simulink model "STLA_8_31"  (R2020b)
settings: Solver=ode3  StartTime=0.0  StopTime=2474  FixedStep=0.01  RelTol=1e-3
model workspace (MAT data in the model file):
  qw = 0.5
undefined symbols (not defined in the file): BSFC, continuous_torque_M, eff_speeds, eff_torques, h, km, m, m_eff, Padd, peak_torque_M, pedal_Brake, pedal_Comfort, pedal_ECO, pedal_Sport, rpm_E, rpm_M, s, speed_bp, speed_Brake, speed_Comfort, speed_ECO, speed_Sport, Tmax_eng, Topt_eng, torque_bp, torque_Brake, Torque_BSFC, torque_Comfort, torque_ECO, torque_Sport
libraries: simulink x12, svdutilitieslib x2, instrumentlib x2, autolibshared x1, aerolibconvert2 x1, pid_lib x1
(part 1 of 2)
settings Model: Creator=王刚  LastModifiedBy=王刚
settings DebuggingCC: UnconnectedInputMsg=none  UnconnectedOutputMsg=none  UnconnectedLineMsg=none
settings ModelReferenceCC: EnableRefExpFcnMdlSchedulingChecks=off
settings RTWCC: GPUComputeCapability=5.0
settings ConfigComp: CovBoundaryAbsTol=1.0e-5

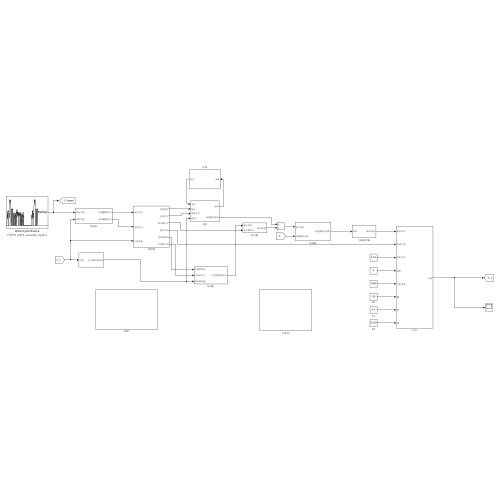
[thumbnail: Simulink's stored preview of the top-level diagram]
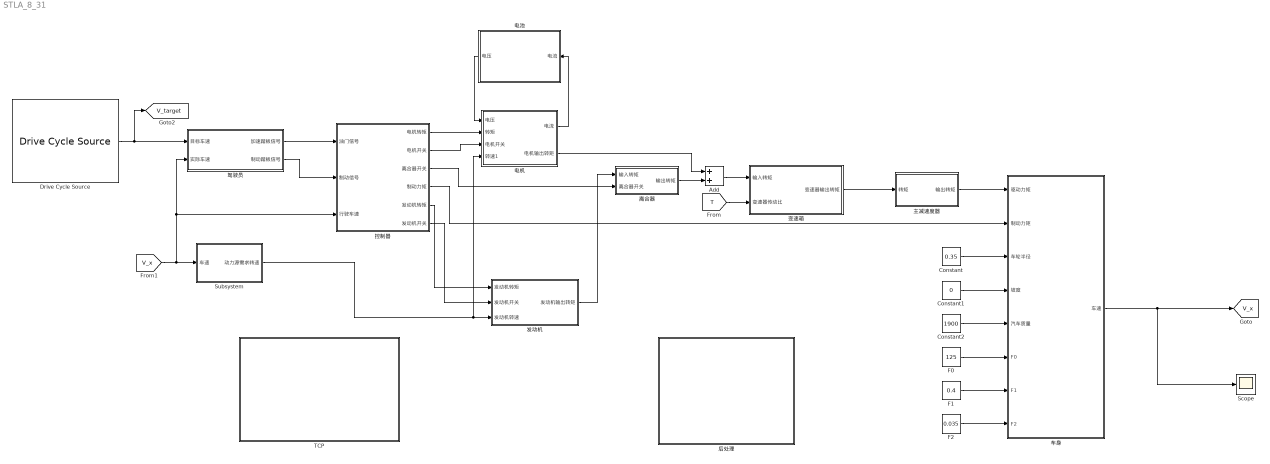
== system STLA_8_31 ==
  Add : Sum
  Constant : Constant  Value=0.35
  Constant1 : Constant  Value=0
  Constant2 : Constant  Value=1900
  Drive Cycle Source : autolibshared/Drive Cycle Source  cycleVar=FTP75  fileVar=cycleFTP75.mat  tfinal="2474  seconds, Cyclic"  cycleRepeat=on  outAccPort=off  outGearPort=off  gearList=No gear data  t_wot1=5  xdot_woto=0  xdot_wot1=30  t_wot2=20  xdot_wot2=0  t_wotend=30  srcUnit=m/s  outUnit=km/h  srcAccUnit=m/s/s  outAccUnit=m/s^2  dt=0  aMode=1  faultOption=off  velBnd=2  velBndUnit=mph  inUnit=m/s  timeBnd=1  failOption=off  stopSim=off  maxFaultCnt=10  maxFaultTime=2  maxTotFaultTime=15  traceOption=off  dtTrace=1  traceWindow=10  lastDCname=FTP75  lastOutUnit=mph  lastDT=0  lastTB=1  lastSB=2  forceCalcBound=off
  F0 : Constant  Value=125
  F1 : Constant  Value=0.4
  F2 : Constant  Value=0.035
  Scope : Scope
  Subsystem : Subsystem
  TCP : Subsystem
  主减速度器 : Subsystem
  发动机 : Subsystem
  变速箱 : Subsystem
  后处理 : Subsystem
  控制器 : Subsystem
  电机 : Subsystem
  电池 : Subsystem
  离合器 : Subsystem
  车身 : Subsystem
  驾驶员 : Subsystem
  tag scope: V_target=global, V_x=global
  wires:
  驾驶员/1(加速踏板信号) -> 控制器/1(油门信号)
  驾驶员/2(制动踏板信号) -> 控制器/2(制动信号)
  Constant/1 -> 车身/3(车轮半径)
  Constant1/1 -> 车身/4(坡度)
  Constant2/1 -> 车身/5(汽车质量)
  F0/1 -> 车身/6(F0)
  F1/1 -> 车身/7(F1)
  F2/1 -> 车身/8(F2)
  变速箱/1(变速器输出转矩) -> 主减速度器/1(转矩)
  主减速度器/1(输出转矩) -> 车身/1("驱动力矩 ")
  控制器/5(发动机转矩) -> 发动机/1(发动机转矩)
  控制器/6(发动机开关) -> 发动机/2(发动机开关)
  控制器/1(电机转矩) -> 电机/2(转矩)
  控制器/2(电机开关) -> 电机/3(电机开关)
  控制器/3(离合器开关) -> 离合器/2(离合器开关)
  控制器/4(制动力矩) -> 车身/2(" 制动力矩")
  电池/1(电压) -> 电机/1(电压)
  离合器/1(输出转矩) -> Add/2
  Add/1 -> 变速箱/1(输入转矩)
  [T] -> 变速箱/2(变速器传动比)
  车身/1(车速) -> [V_x], Scope/1
  [V_x] -> 驾驶员/2(实际车速), 控制器/3(行驶车速), Subsystem/1(车速)
  电机/1(电流) -> 电池/1(电流)
  电机/2(电机输出转矩) -> Add/1
  发动机/1(发动机输出转矩) -> 离合器/1(输入转矩)
  Subsystem/1(动力源需求转速) -> 电机/4(转速1), 发动机/3(发动机转速)
  Drive Cycle Source/1 -> [V_target], 驾驶员/1(目标车速)

== system STLA_8_31/Subsystem ==
  车速 : Inport
  " " : Constant  Value=0.377
  Product : Product  Inputs=***//
  主减速器传动比 : Constant  Value=4.88
  车轮半径 : Constant  Value=0.25
  动力源需求转速 : Outport
  tag scope: rmp=global
  wires:
  Product/1 -> [rmp], 动力源需求转速/1
  车速/1 -> Product/1
  " "/1 -> Product/5
  主减速器传动比/1 -> Product/2
  车轮半径/1 -> Product/4
  [T] -> Product/3

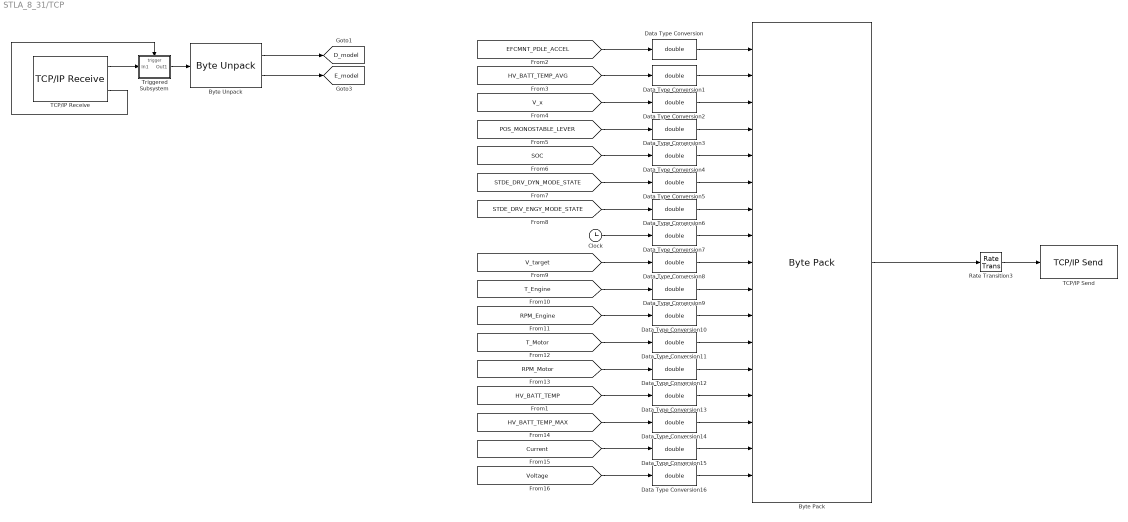
== system STLA_8_31/TCP ==
  Byte Pack : svdutilitieslib/Byte Pack  maskPackedDataType=uint8  datatypes={'double', 'double', 'double', 'double', 'double', 'double', 'double', 'double', 'double', 'double', 'double', 'double', 'double', 'double', 'double', 'double', 'double'}  byteAlign=1  blockPlatform=tic2000
  Byte Unpack : svdutilitieslib/Byte Unpack  dimensions={[1] [1]}  datatypes={'double', 'double'}  byteAlign=1  blockPlatform=tic2000
  Clock : Clock
  Data Type Conversion{,1..16} (17 alike) : DataTypeConversion  OutDataTypeStr=double
  Rate Transition3 : RateTransition  OutPortSampleTime=0.1
  TCP/IP Receive : instrumentlib/TCP//IP Receive  Host=127.0.0.1  Port=5000  DataSize=16  DataType=uint8  ASCIIFormatting=%f  Terminator=LF  ByteOrder=LittleEndian  EnableBlockingMode=off  Timeout=0.01  SampleTime=0.01
  TCP/IP Send : instrumentlib/TCP//IP Send  Host=127.0.0.1  Port=5001  ByteOrder=LittleEndian  EnableBlockingMode=off  Timeout=10  TransferDelay=on
  Triggered Subsystem : Subsystem  TreatAsAtomicUnit=on
  tag scope: D_model=global, E_model=global
  wires:
  [SOC] -> Data Type Conversion4/1
  [V_x] -> Data Type Conversion2/1
  Byte Unpack/2 -> [E_model]
  Data Type Conversion1/1 -> Byte Pack/2
  Data Type Conversion8/1 -> Byte Pack/9
  Data Type Conversion6/1 -> Byte Pack/7
  [V_target] -> Data Type Conversion8/1
  [EFCMNT_PDLE_ACCEL] -> Data Type Conversion/1
  [RPM_Engine] -> Data Type Conversion10/1
  [STDE_DRV_DYN_MODE_STATE] -> Data Type Conversion5/1
  Data Type Conversion12/1 -> Byte Pack/13
  Data Type Conversion3/1 -> Byte Pack/4
  [T_Engine] -> Data Type Conversion9/1
  Data Type Conversion10/1 -> Byte Pack/11
  Data Type Conversion5/1 -> Byte Pack/6
  Data Type Conversion11/1 -> Byte Pack/12
  Byte Pack/1 -> Rate Transition3/1
  TCP/IP Receive/2 -> Triggered Subsystem/Trigger
  TCP/IP Receive/1 -> Triggered Subsystem/1(In1)
  [T_Motor] -> Data Type Conversion11/1
  Triggered Subsystem/1(Out1) -> Byte Unpack/1
  Data Type Conversion4/1 -> Byte Pack/5
  Byte Unpack/1 -> [D_model]
  [POS_MONOSTABLE_LEVER] -> Data Type Conversion3/1
  [RPM_Motor] -> Data Type Conversion12/1
  Data Type Conversion2/1 -> Byte Pack/3
  [STDE_DRV_ENGY_MODE_STATE] -> Data Type Conversion6/1
  Clock/1 -> Data Type Conversion7/1
  Data Type Conversion7/1 -> Byte Pack/8
  Rate Transition3/1 -> TCP/IP Send/1
  [HV_BATT_TEMP_AVG] -> Data Type Conversion1/1
  Data Type Conversion9/1 -> Byte Pack/10
  Data Type Conversion/1 -> Byte Pack/1
  [HV_BATT_TEMP] -> Data Type Conversion13/1
  [HV_BATT_TEMP_MAX] -> Data Type Conversion14/1
  Data Type Conversion13/1 -> Byte Pack/14
  Data Type Conversion14/1 -> Byte Pack/15
  [Current] -> Data Type Conversion15/1
  [Voltage] -> Data Type Conversion16/1
  Data Type Conversion15/1 -> Byte Pack/16
  Data Type Conversion16/1 -> Byte Pack/17

== system STLA_8_31/主减速度器 ==
  转矩 : Inport
  Product : Product
  主减速器传动比 : Constant  Value=4.88
  传动效率 : Gain  Gain=0.9
  输出转矩 : Outport
  wires:
  转矩/1 -> Product/1
  主减速器传动比/1 -> Product/2
  Product/1 -> 传动效率/1
  传动效率/1 -> 输出转矩/1

== system STLA_8_31/发动机 ==
  发动机转矩 : Inport
  发动机开关 : Inport  Port=2
  发动机转速 : Inport  Port=3
  2-D Lookup Table : Lookup_n-D  BreakpointsForDimension1=Torque_BSFC  BreakpointsForDimension2=rpm_E  Table=BSFC  InternalRulePriority=Speed  RndMeth=Simplest  InputSameDT=on
      settings: InputPortMap=u0,u1
  Constant : Constant  Value=9550
  Constant1 : Constant  Value=3600
  Gain : Gain  Gain=-1
  Integrator : Integrator
  Product : Product
  Product1 : Product  Inputs=***/
  Product2 : Product  Inputs=**/
  Product3 : Product
  Saturation Dynamic : simulink/Discontinuities/Saturation Dynamic  OutMin=[]  OutMax=[]  OutDataTypeStr=Inherit: Same as second input  OutDataType=fixdt(1, 16)  OutScaling=2^-10  DoSatur=off
  Scope : Scope
  Scope2 : Scope  NumInputPorts=3
  Scope3 : Scope  NumInputPorts=2
  外特性 : Lookup_n-D  NumberOfTableDimensions=1  BreakpointsForDimension1=rpm_E  Table=Tmax_eng  InternalRulePriority=Speed  RndMeth=Simplest  InputSameDT=on
  最优转矩 : Lookup_n-D  NumberOfTableDimensions=1  BreakpointsForDimension1=rpm_E  Table=Topt_eng  InternalRulePriority=Speed  RndMeth=Simplest  InputSameDT=on
  发动机输出转矩 : Outport
  tag scope: M_f=global, RPM_Engine=global, T_Engine=global, Te_max=global, Te_opt=global
  wires:
  Constant/1 -> Product1/4
  Product1/1 -> Product2/1, Scope/1
  发动机开关/1 -> Product3/2, Product1/3, Scope2/2, Product/1
  最优转矩/1 -> Scope3/2, [Te_opt]
  外特性/1 -> Gain/1, Scope3/1, Saturation Dynamic/1, [Te_max]
  发动机转矩/1 -> 2-D Lookup Table/1, Product1/2, Scope2/3, Product/2
  Saturation Dynamic/1 -> Scope2/1, 发动机输出转矩/1, [T_Engine]
  Product/1 -> Saturation Dynamic/2
  Gain/1 -> Saturation Dynamic/3
  2-D Lookup Table/1 -> Product2/2
  Constant1/1 -> Product2/3
  Product2/1 -> Integrator/1
  Integrator/1 -> [M_f]
  发动机转速/1 -> Product3/1, 最优转矩/1, 2-D Lookup Table/2, Product1/1, 外特性/1
  Product3/1 -> [RPM_Engine]

== system STLA_8_31/变速箱 ==
  输入转矩 : Inport
  变速器传动比 : Inport  Port=2
  Product : Product
  变速器输出转矩 : Outport
  wires:
  输入转矩/1 -> Product/1
  变速器传动比/1 -> Product/2
  Product/1 -> 变速器输出转矩/1

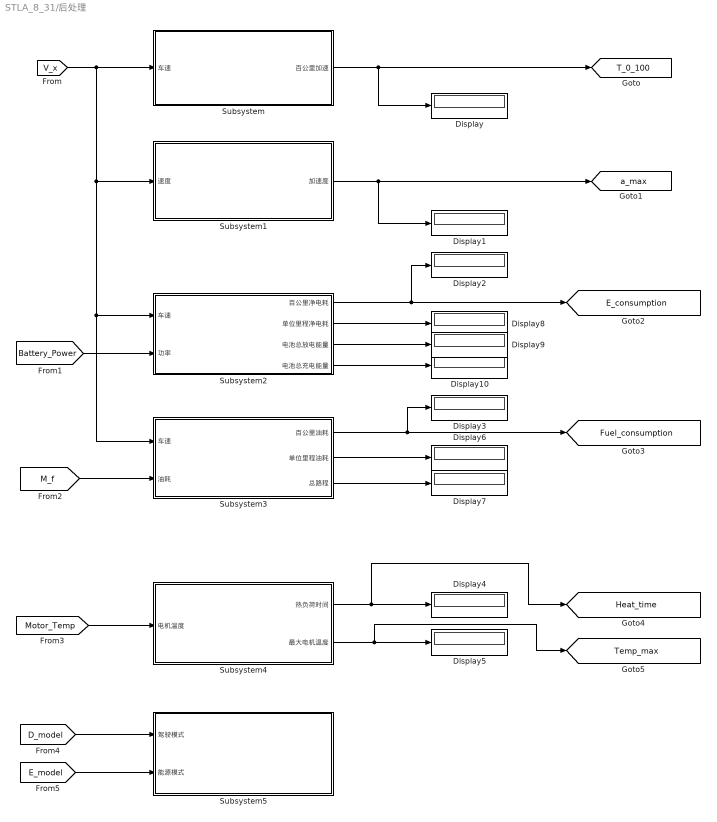
== system STLA_8_31/后处理 ==
  Display{,1..10} (11 alike) : Display
  Subsystem : Subsystem
  Subsystem1 : Subsystem
  Subsystem2 : Subsystem
  Subsystem3 : Subsystem
  Subsystem4 : Subsystem
  Subsystem5 : Subsystem
  tag scope: E_consumption=global, Fuel_consumption=global, Heat_time=global, T_0_100=global, Temp_max=global, a_max=global
  wires:
  [V_x] -> Subsystem2/1(车速), Subsystem3/1(车速), Subsystem1/1(速度), Subsystem/1(车速)
  Subsystem2/1(百公里净电耗) -> Display2/1, [E_consumption]
  [Battery_Power] -> Subsystem2/2(功率)
  [M_f] -> Subsystem3/2(油耗)
  Subsystem3/1(百公里油耗) -> [Fuel_consumption], Display3/1
  [Motor_Temp] -> Subsystem4/1(电机温度)
  Subsystem4/1(热负荷时间) -> [Heat_time], Display4/1
  [D_model] -> Subsystem5/1(驾驶模式)
  Subsystem/1(百公里加速) -> Display/1, [T_0_100]
  Subsystem1/1(加速度) -> Display1/1, [a_max]
  Subsystem4/2(最大电机温度) -> [Temp_max], Display5/1
  [E_model] -> Subsystem5/2(能源模式)
  Subsystem3/2(单位里程油耗) -> Display6/1
  Subsystem3/3(总路程) -> Display7/1
  Subsystem2/2(单位里程净电耗) -> Display8/1
  Subsystem2/3(电池总放电能量) -> Display9/1
  Subsystem2/4(电池总充电能量) -> Display10/1

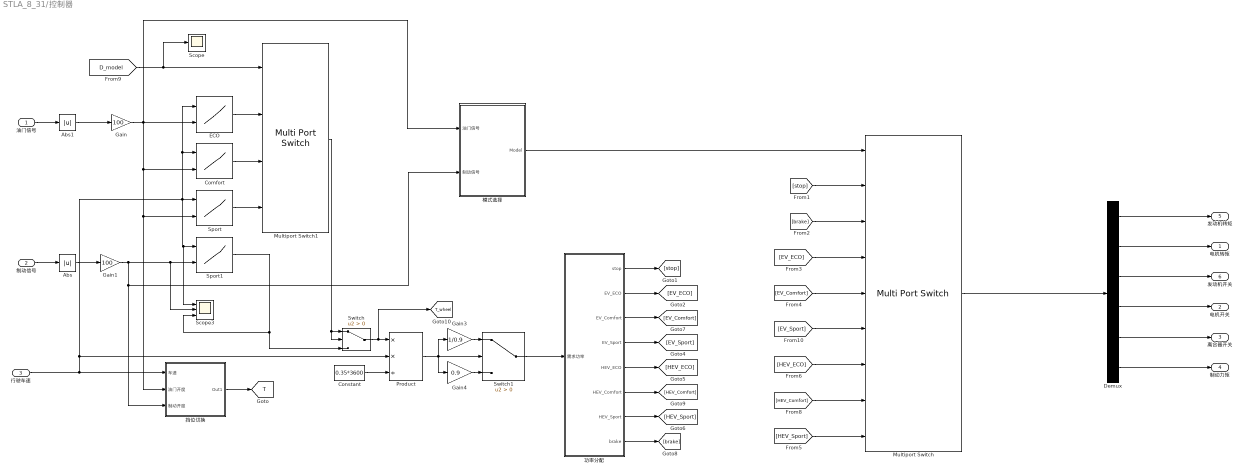
== system STLA_8_31/控制器 ==
  油门信号 : Inport
  制动信号 : Inport  Port=2
  行驶车速 : Inport  Port=3
  Abs : Abs  ZeroCross=off
  Abs1 : Abs  ZeroCross=off
  Comfort : Lookup_n-D  BreakpointsForDimension1=speed_Comfort  BreakpointsForDimension2=pedal_Comfort  Table=torque_Comfort  InternalRulePriority=Speed  RndMeth=Simplest  InputSameDT=on
      settings: InputPortMap=u0,u1
  Constant : Constant  Value=0.35*3600
  Demux : Demux  Outputs=6
  ECO : Lookup_n-D  BreakpointsForDimension1=speed_ECO  BreakpointsForDimension2=pedal_ECO  Table=torque_ECO  InternalRulePriority=Speed  RndMeth=Simplest  InputSameDT=on
      settings: InputPortMap=u0,u1
  Gain : Gain  Gain=100
  Gain1 : Gain  Gain=100
  Gain3 : Gain  Gain=1/0.9
  Gain4 : Gain  Gain=0.9
  Multiport Switch : MultiPortSwitch  Inputs=8
  Multiport Switch1 : MultiPortSwitch  DataPortOrder=Zero-based contiguous  DiagnosticForDefault=None  zeroidx=on
  Product : Product  Inputs=**/
  Scope : Scope
  Scope3 : Scope  NumInputPorts=3
  Sport : Lookup_n-D  BreakpointsForDimension1=speed_Sport  BreakpointsForDimension2=pedal_Sport  Table=torque_Sport  InternalRulePriority=Speed  RndMeth=Simplest  InputSameDT=on
      settings: InputPortMap=u0,u1
  Sport1 : Lookup_n-D  BreakpointsForDimension1=speed_Brake  BreakpointsForDimension2=pedal_Brake  Table=torque_Brake  InternalRulePriority=Speed  RndMeth=Simplest  InputSameDT=on
      settings: InputPortMap=u0,u1
  Switch : Switch  Criteria=u2 > Threshold  ZeroCross=off
  Switch1 : Switch  Criteria=u2 > Threshold
  功率分配 : Subsystem
  挡位切换 : Subsystem
  模式选择 : Subsystem
  电机转矩 : Outport
  电机开关 : Outport  Port=2
  离合器开关 : Outport  Port=3
  制动力矩 : Outport  Port=4
  发动机转矩 : Outport  Port=5
  发动机开关 : Outport  Port=6
  tag scope: T=global, T_wheel=global
  wires:
  油门信号/1 -> Abs1/1
  制动信号/1 -> Abs/1
  Abs/1 -> Gain1/1
  Sport1/1 -> Scope3/3, Switch/3
  ECO/1 -> Multiport Switch1/2
  行驶车速/1 -> Product/2, Scope3/1, Sport1/1, ECO/1, Comfort/1, Sport/1, 挡位切换/1(车速)
  功率分配/1(stop) -> [stop]
  功率分配/2(EV_ECO) -> [EV_ECO]
  [stop] -> Multiport Switch/2
  [brake] -> Multiport Switch/3
  [EV_Comfort] -> Multiport Switch/5
  [EV_Sport] -> Multiport Switch/6
  [HEV_ECO] -> Multiport Switch/7
  [EV_ECO] -> Multiport Switch/4
  Multiport Switch/1 -> Demux/1
  Demux/1 -> 发动机转矩/1
  Demux/2 -> 电机转矩/1
  Demux/3 -> 发动机开关/1
  Demux/4 -> 电机开关/1
  Demux/5 -> 离合器开关/1
  Demux/6 -> 制动力矩/1
  模式选择/1(Model) -> Multiport Switch/1
  功率分配/3(EV_Comfort) -> [EV_Comfort]
  功率分配/4(EV_Sport) -> [EV_Sport]
  功率分配/5(HEV_ECO) -> [HEV_ECO]
  功率分配/7(HEV_Sport) -> [HEV_Sport]
  功率分配/6(HEV_Comfort) -> [HEV_Comfort]
  功率分配/8(brake) -> [brake]
  [HEV_Comfort] -> Multiport Switch/8
  [HEV_Sport] -> Multiport Switch/9
  挡位切换/1(Out1) -> [T]
  Comfort/1 -> Multiport Switch1/3
  Sport/1 -> Multiport Switch1/4
  [D_model] -> Scope/1, Multiport Switch1/1
  Abs1/1 -> Gain/1
  Gain/1 -> 模式选择/1(油门信号), ECO/2, Comfort/2, Sport/2, 挡位切换/2(油门开度)
  Gain1/1 -> Scope3/2, Sport1/2, 模式选择/2(制动信号), 挡位切换/3(制动开度)
  Switch/1 -> [T_wheel], Product/1
  Constant/1 -> Product/3
  Gain3/1 -> Switch1/1
  Gain4/1 -> Switch1/3
  Switch1/1 -> 功率分配/1(需求功率)
  Product/1 -> Gain3/1, Gain4/1, Switch1/2
  Multiport Switch1/1 -> Switch/2, Switch/1

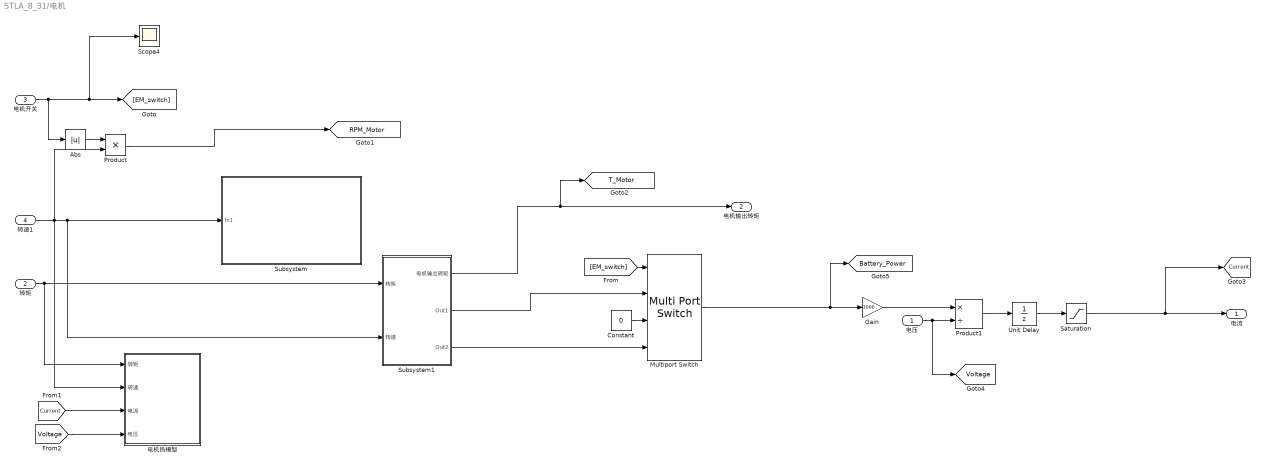
== system STLA_8_31/电机 ==
  电压 : Inport
  转矩 : Inport  Port=2
  电机开关 : Inport  Port=3
  转速1 : Inport  Port=4
  Abs : Abs
  Constant : Constant  Value=0
  Gain : Gain  Gain=1000
  Multiport Switch : MultiPortSwitch  DataPortOrder=Specify indices  DataPortIndices={1,0,-1}
  Product : Product
  Product1 : Product  Inputs=*/
  Saturation : Saturate  UpperLimit=250  LowerLimit=-250  ZeroCross=off
  Scope4 : Scope
  Subsystem : Subsystem
  Subsystem1 : Subsystem
  Unit Delay : UnitDelay  SampleTime=-1  HasFrameUpgradeWarning=on
  电机热模型 : Subsystem
  电流 : Outport
  电机输出转矩 : Outport  Port=2
  tag scope: Battery_Power=global, Current=global, RPM_Motor=global, T_Motor=global, Voltage=global
  wires:
  Gain/1 -> Product1/1
  电压/1 -> [Voltage], Product1/2
  Product1/1 -> Unit Delay/1
  Unit Delay/1 -> Saturation/1
  转速1/1 -> Product/2, Subsystem/1(In1), Subsystem1/2(转速), 电机热模型/2(转速)
  Constant/1 -> Multiport Switch/3
  电机开关/1 -> Abs/1, Scope4/1, [EM_switch]
  [EM_switch] -> Multiport Switch/1
  Multiport Switch/1 -> [Battery_Power], Gain/1
  转矩/1 -> 电机热模型/1(转矩), Subsystem1/1(转矩)
  [Current] -> 电机热模型/3(电流)
  [Voltage] -> 电机热模型/4(电压)
  Subsystem1/2(Out1) -> Multiport Switch/2
  Subsystem1/3(Out2) -> Multiport Switch/4
  Subsystem1/1(电机输出转矩) -> [T_Motor], 电机输出转矩/1
  Product/1 -> [RPM_Motor]
  Abs/1 -> Product/1
  Saturation/1 -> [Current], 电流/1

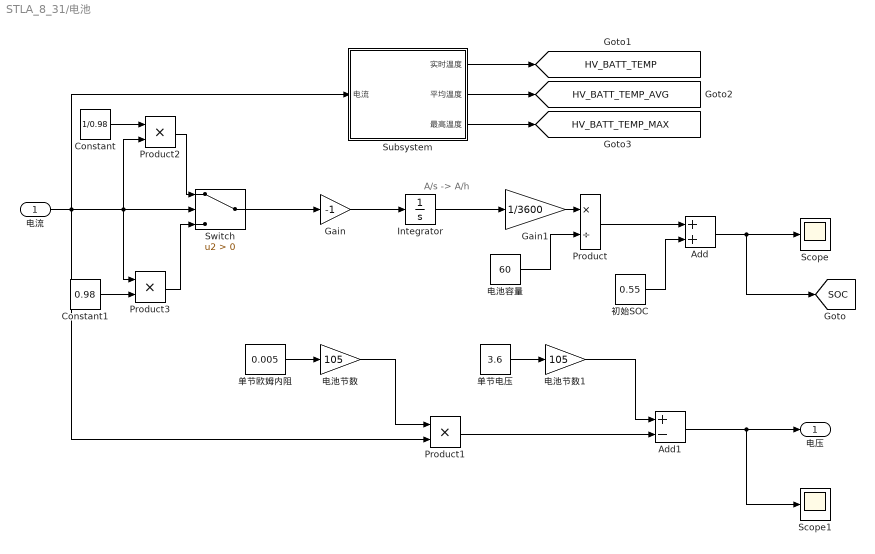
== system STLA_8_31/电池 ==
  note: A/s -> A/h
  电流 : Inport
  Add : Sum
  Add1 : Sum  Inputs=+-
  Constant : Constant  Value=1/0.98
  Constant1 : Constant  Value=0.98
  Gain : Gain  Gain=-1
  Gain1 : Gain  Gain=1/3600
  Integrator : Integrator
  Product : Product  Inputs=*/
  Product1 : Product
  Product2 : Product
  Product3 : Product
  Scope : Scope
  Scope1 : Scope
  Subsystem : Subsystem
  Switch : Switch  Criteria=u2 > Threshold
  初始SOC : Constant  Value=0.55
  单节欧姆内阻 : Constant  Value=0.005
  单节电压 : Constant  Value=3.6
  电池容量 : Constant  Value=60
  电池节数 : Gain  Gain=105
  电池节数1 : Gain  Gain=105
  电压 : Outport
  tag scope: HV_BATT_TEMP=global, HV_BATT_TEMP_AVG=global, HV_BATT_TEMP_MAX=global, SOC=global
  wires:
  Gain/1 -> Integrator/1
  Integrator/1 -> Gain1/1
  Gain1/1 -> Product/1
  电池容量/1 -> Product/2
  Product/1 -> Add/1
  初始SOC/1 -> Add/2
  Add/1 -> [SOC], Scope/1
  电流/1 -> Product3/1, Product2/2, Switch/2, Subsystem/1(电流), Product1/2
  单节欧姆内阻/1 -> 电池节数/1
  电池节数/1 -> Product1/1
  单节电压/1 -> 电池节数1/1
  电池节数1/1 -> Add1/1
  Product1/1 -> Add1/2
  Add1/1 -> Scope1/1, 电压/1
  Subsystem/1(实时温度) -> [HV_BATT_TEMP]
  Switch/1 -> Gain/1
  Constant/1 -> Product2/1
  Product2/1 -> Switch/1
  Constant1/1 -> Product3/2
  Product3/1 -> Switch/3
  Subsystem/3(最高温度) -> [HV_BATT_TEMP_MAX]
  Subsystem/2(平均温度) -> [HV_BATT_TEMP_AVG]

== system STLA_8_31/离合器 ==
  输入转矩 : Inport
  离合器开关 : Inport  Port=2
  Product : Product
  输出转矩 : Outport
  wires:
  输入转矩/1 -> Product/1
  离合器开关/1 -> Product/2
  Product/1 -> 输出转矩/1

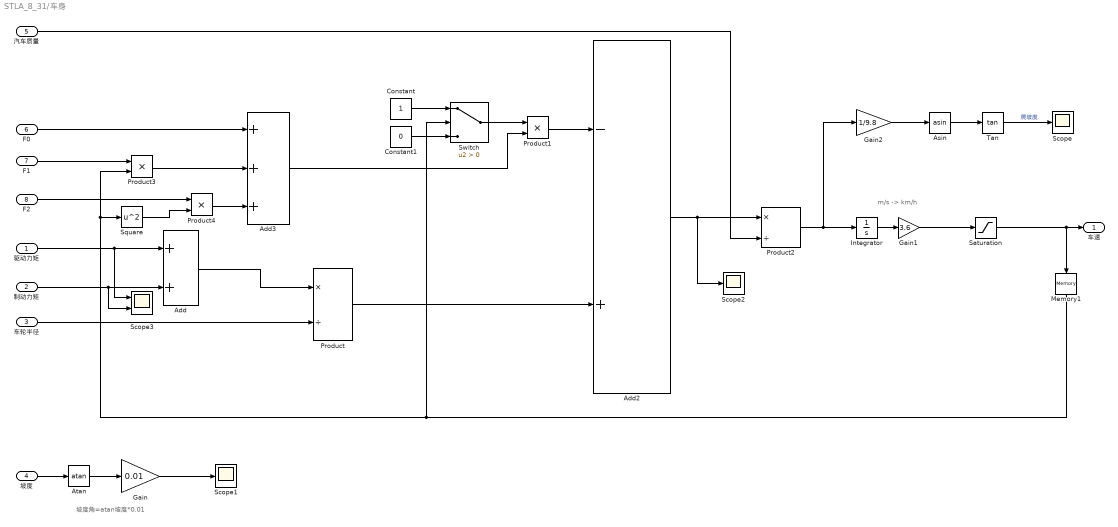
== system STLA_8_31/车身 ==
  note: m/s -> km/h
  note: 坡度角=atan坡度*0.01
  "驱动力矩 " : Inport
  " 制动力矩" : Inport  Port=2
  车轮半径 : Inport  Port=3
  坡度 : Inport  Port=4
  汽车质量 : Inport  Port=5
  F0 : Inport  Port=6
  F1 : Inport  Port=7
  F2 : Inport  Port=8
  Add : Sum
  Add2 : Sum  Inputs=-+
  Add3 : Sum  Inputs=+++
  Asin : Trigonometry  Operator=asin
  Atan : Trigonometry  Operator=atan
  Constant : Constant
  Constant1 : Constant  Value=0
  Gain : Gain  Gain=0.01
  Gain1 : Gain  Gain=3.6
  Gain2 : Gain  Gain=1/9.8
  Integrator : Integrator  ZeroCross=off
  Memory1 : Memory
  Product : Product  Inputs=*/
  Product1 : Product
  Product2 : Product  Inputs=*/
  Product3 : Product
  Product4 : Product
  Saturation : Saturate  UpperLimit=100000  LowerLimit=0  ZeroCross=off
  Scope : Scope
  Scope1 : Scope
  Scope2 : Scope
  Scope3 : Scope  NumInputPorts=2
  Square : Math  Operator=square  SaturateOnIntegerOverflow=on
  Switch : Switch  Criteria=u2 > Threshold
  Tan : Trigonometry  Operator=tan
  车速 : Outport
  wires:
  "驱动力矩 "/1 -> Scope3/1, Add/1
  " 制动力矩"/1 -> Scope3/2, Add/2
  Add/1 -> Product/1
  车轮半径/1 -> Product/2
  坡度/1 -> Atan/1
  Atan/1 -> Gain/1
  汽车质量/1 -> Product2/2
  Switch/1 -> Product1/1
  Constant/1 -> Switch/1
  Constant1/1 -> Switch/3
  Product1/1 -> Add2/1
  Product/1 -> Add2/2
  Add2/1 -> Scope2/1, Product2/1
  Product2/1 -> Gain2/1, Integrator/1
  Add3/1 -> Product1/2
  Gain2/1 -> Asin/1
  Asin/1 -> Tan/1
  Tan/1 -> Scope/1  "爬坡度"
  Gain/1 -> Scope1/1
  F0/1 -> Add3/1
  F1/1 -> Product3/1
  F2/1 -> Product4/1
  Integrator/1 -> Gain1/1
  Square/1 -> Product4/2
  Product3/1 -> Add3/2
  Product4/1 -> Add3/3
  Saturation/1 -> 车速/1, Memory1/1
  Gain1/1 -> Saturation/1
  Memory1/1 -> Square/1, Product3/2, Switch/2

== system STLA_8_31/驾驶员 ==
  目标车速 : Inport
  实际车速 : Inport  Port=2
  Constant : Constant  Value=0
  Constant1 : Constant  Value=0.01
  PID Controller : pid_lib/PID Controller  Controller=PI  Form=Parallel  TimeDomain=Continuous-time  UseExternalTs=off  SampleTime=-1  IntegratorMethod=Forward Euler  ControllerParametersSource=internal  P=0.5  I=0.06  D=0  N=100  UseFilter=on  TunerSelectOption=Transfer Function Based (PID Tuner App)  InitialConditionSource=internal  InitialConditionForIntegrator=0  InitialConditionForFilter=0  DifferentiatorICPrevScaledInput=0  ExternalReset=falling  TrackingMode=off  Kt=1  LimitOutput=off  SatLimitsSource=internal  UpperSaturationLimit=inf  LowerSaturationLimit=-inf  LinearizeAsGain=on  AntiWindupMode=none  Kb=1  POutMin=[]  POutMax=[]  IOutMin=[]  IOutMax=[]  DOutMin=[]  DOutMax=[]  NOutMin=[]  NOutMax=[]  SumOutMin=[]  SumOutMax=[]  SaturationOutMin=[]  SaturationOutMax=[]  PParamMin=[]  PParamMax=[]  IParamMin=[]  IParamMax=[]  DParamMin=[]  DParamMax=[]  NParamMin=[]  NParamMax=[]  KbParamMin=[]  KbParamMax=[]  KtParamMin=[]  KtParamMax=[]  KbOutMin=[]  KbOutMax=[]  KtOutMin=[]  KtOutMax=[]  IntegratorOutMin=[]  IntegratorOutMax=[]  FilterOutMin=[]  FilterOutMax=[]  SumI1OutMin=[]  SumI1OutMax=[]  SumI2OutMin=[]  SumI2OutMax=[]  SumI3OutMin=[]  SumI3OutMax=[]  SumI4OutMin=[]  SumI4OutMax=[]  SumDOutMin=[]  SumDOutMax=[]  DifferentiatorOutMin=[]  DifferentiatorOutMax=[]  FilterDiffOutCoefMin=[]  FilterDiffOutCoefMax=[]  ReciprocalOutMin=[]  ReciprocalOutMax=[]  SumDenOutMin=[]  SumDenOutMax=[]  SumNumOutMin=[]  SumNumOutMax=[]  DivideOutMin=[]  DivideOutMax=[]  UdiffTsProdOutMin=[]  UdiffTsProdOutMax=[]  NTsProdOutMin=[]  NTsProdOutMax=[]  UintegralTsProdOutMin=[]  UintegralTsProdOutMax=[]  UngainTsProdOutMin=[]  UngainTsProdOutMax=[]  IntegratorContinuousStateAttributes=''  IntegratorStateMustResolveToSignalObject=off  IntegratorRTWStateStorageClass=Auto  FilterContinuousStateAttributes=''  FilterStateMustResolveToSignalObject=off  FilterRTWStateStorageClass=Auto  ParallelPVariant=InternalParameters  IdealPVariant=Disabled  IVariant=InternalParameters  DVariant=Disabled  IntegratorVariant=Continuous  SatVariant=Disabled  AWVariant=Passthrough  PCopyVariant=Disabled  TRVariant=Disabled  FdbkBlocksVariant=Forward  IdealPFdbkVariant=Disabled  SatFdbkVariant=Disabled  DerivativeFilterVariant=Disabled  NVariant=Disabled  NCopyVariant=Disabled_SignalSpec  FilterICVariant=Disabled  IntegratorICVariant=InternalICs  ExternalResetVariant=ExternalReset  TRSumVariant=Passthrough  SumFdbkVariant=Disabled  SumVariant=Sum_PI  TsampFilterVariant=InternalTs  TsampNgainVariant=Passthrough  TsampIntegralVariant=Disabled_SignalSpec  ExternalSaturationOutDataTypeStr=Inherit: Same as second input
  Relational Operator : RelationalOperator  OutDataTypeStr=boolean  RndMeth=Simplest
  Saturation : Saturate  UpperLimit=1  LowerLimit=-1
  Sum : Sum  Inputs=|+-
  Switch : Switch  Criteria=u2 > Threshold  ZeroCross=off
  Switch1 : Switch  Criteria=u2 > Threshold  ZeroCross=off
  加速踏板信号 : Outport
  制动踏板信号 : Outport  Port=2
  tag scope: EFCMNT_PDLE_ACCEL=global
  wires:
  目标车速/1 -> Sum/1
  实际车速/1 -> Sum/2, Relational Operator/1
  Sum/1 -> PID Controller/1
  PID Controller/1 -> Saturation/1
  Saturation/1 -> Switch1/3, Switch1/2, Switch/2, Switch/1
  Switch/1 -> [EFCMNT_PDLE_ACCEL], 加速踏板信号/1
  Switch1/1 -> 制动踏板信号/1
  Constant/1 -> Switch/3, Switch1/1
  Relational Operator/1 -> PID Controller/2
  Constant1/1 -> Relational Operator/2

== system STLA_8_31/TCP/Triggered Subsystem ==
  In1 : Inport
  Trigger : TriggerPort  VariantControl=(inherit)
  Out1 : Outport
  wires:
  In1/1 -> Out1/1

== system STLA_8_31/后处理/Subsystem ==
  车速 : Inport
  AND : Logic  IconShape=distinctive  AllPortsSameDT=off  OutDataTypeStr=boolean
  Clock : Clock
  Compare To Constant : simulink/Logic and Bit Operations/Compare To Constant  relop=>=  const=100  OutDataTypeStr=boolean
  Constant : Constant  Value=0
  Detect Rise Positive : simulink/Logic and Bit Operations/Detect Rise Positive  vinit=0  OutDataTypeStr=boolean
  Triggered Subsystem : Subsystem  TreatAsAtomicUnit=on
  百公里加速 : Outport
  wires:
  车速/1 -> Compare To Constant/1
  Constant/1 -> AND/2
  Triggered Subsystem/1(Out1) -> 百公里加速/1
  Compare To Constant/1 -> AND/1
  Detect Rise Positive/1 -> Triggered Subsystem/Trigger
  Clock/1 -> Triggered Subsystem/1(In1)
  AND/1 -> Detect Rise Positive/1

== system STLA_8_31/后处理/Subsystem1 ==
  速度 : Inport
  Acceleration Conversion : aerolibconvert2/Acceleration Conversion  IU=m/s^2  OU=km/h-s
  Derivative : Derivative
  Gain : Gain  Gain=1/3.6
  Memory : Memory
  MinMax : MinMax  Function=max  Inputs=2
  Saturation : Saturate  UpperLimit=inf  LowerLimit=0
  加速度 : Outport
  wires:
  Acceleration Conversion/1 -> Saturation/1
  Gain/1 -> Derivative/1
  Derivative/1 -> Acceleration Conversion/1
  速度/1 -> Gain/1
  MinMax/1 -> 加速度/1, Memory/1
  Saturation/1 -> MinMax/1
  Memory/1 -> MinMax/2

== system STLA_8_31/后处理/Subsystem2 ==
  车速 : Inport
  功率 : Inport  Port=2
  Constant : Constant  Value=0
  Constant1 : Constant  Value=0
  Divide : Product  Inputs=*/
  Gain : Gain  Gain=1/3600
  Gain1 : Gain  Gain=1/3.6
  Gain2 : Gain  Gain=1/1000
  Gain3 : Gain  Gain=100
  Gain4 : Gain  Gain=1/3600
  Gain5 : Gain  Gain=1/3600
  Gain6 : Gain  Gain=-1
  Integrator{,1..3} (4 alike) : Integrator
  Max : MinMax  Function=max  Inputs=2
  Max1 : MinMax  Function=max  Inputs=2
  百公里净电耗 : Outport
  单位里程净电耗 : Outport  Port=2
  电池总放电能量 : Outport  Port=3
  电池总充电能量 : Outport  Port=4
  wires:
  Integrator/1 -> Gain/1
  车速/1 -> Gain1/1
  Gain1/1 -> Integrator1/1
  Integrator1/1 -> Gain2/1
  Gain/1 -> Divide/1
  Gain2/1 -> Divide/2
  Divide/1 -> 单位里程净电耗/1, Gain3/1
  Gain3/1 -> 百公里净电耗/1
  Constant/1 -> Max/2
  Max/1 -> Integrator2/1
  Integrator2/1 -> Gain4/1
  Gain4/1 -> 电池总放电能量/1
  Gain5/1 -> 电池总充电能量/1
  Integrator3/1 -> Gain5/1
  Max1/1 -> Integrator3/1
  Constant1/1 -> Max1/2
  功率/1 -> Gain6/1, Max/1, Integrator/1
  Gain6/1 -> Max1/1

== system STLA_8_31/后处理/Subsystem3 ==
  车速 : Inport
  油耗 : Inport  Port=2
  Divide : Product  Inputs=*/
  Gain : Gain  Gain=1/(1000*0.74)
  Gain1 : Gain  Gain=1/3.6
  Gain2 : Gain  Gain=1/1000
  Gain3 : Gain  Gain=100
  Integrator1 : Integrator
  百公里油耗 : Outport
  单位里程油耗 : Outport  Port=2
  总路程 : Outport  Port=3
  wires:
  Gain1/1 -> Integrator1/1
  车速/1 -> Gain1/1
  Integrator1/1 -> Gain2/1
  油耗/1 -> Gain/1
  Divide/1 -> 单位里程油耗/1, Gain3/1
  Gain/1 -> Divide/1
  Gain2/1 -> 总路程/1, Divide/2
  Gain3/1 -> 百公里油耗/1

== system STLA_8_31/后处理/Subsystem4 ==
  电机温度 : Inport
  Compare To Constant : simulink/Logic and Bit Operations/Compare To Constant  relop=>=  const=100  OutDataTypeStr=boolean
  Constant : Constant
  Constant1 : Constant  Value=0
  Integrator : Integrator
  Max : MinMax  Function=max  Inputs=2
  Memory : Memory
  Switch : Switch  Criteria=u2 > Threshold
  热负荷时间 : Outport
  最大电机温度 : Outport  Port=2
  wires:
  电机温度/1 -> Max/1, Compare To Constant/1
  Compare To Constant/1 -> Switch/2
  Constant/1 -> Switch/1
  Constant1/1 -> Switch/3
  Switch/1 -> Integrator/1
  Integrator/1 -> 热负荷时间/1
  Max/1 -> 最大电机温度/1, Memory/1
  Memory/1 -> Max/2

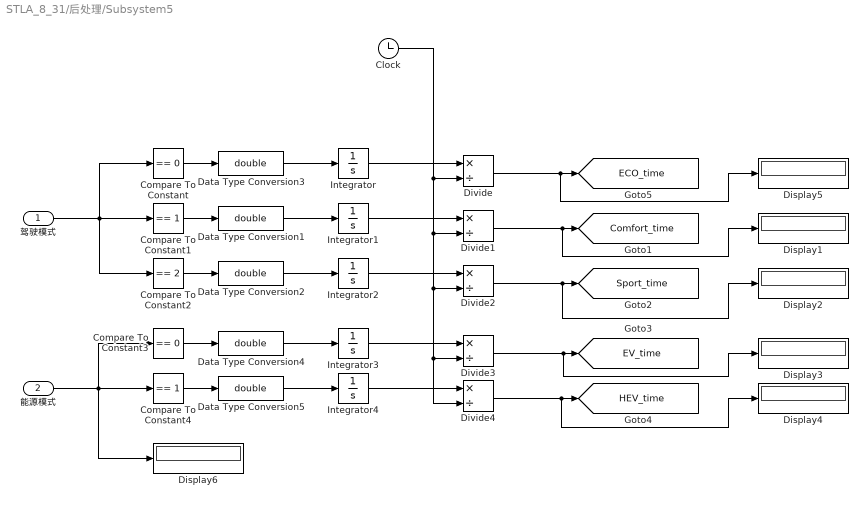
== system STLA_8_31/后处理/Subsystem5 ==
  驾驶模式 : Inport
  能源模式 : Inport  Port=2
  Clock : Clock
  Compare To Constant : simulink/Logic and Bit Operations/Compare To Constant  relop===  const=0  OutDataTypeStr=boolean
  Compare To Constant1 : simulink/Logic and Bit Operations/Compare To Constant  relop===  const=1  OutDataTypeStr=boolean
  Compare To Constant2 : simulink/Logic and Bit Operations/Compare To Constant  relop===  const=2  OutDataTypeStr=boolean
  Compare To Constant3 : simulink/Logic and Bit Operations/Compare To Constant  relop===  const=0  OutDataTypeStr=boolean
  Compare To Constant4 : simulink/Logic and Bit Operations/Compare To Constant  relop===  const=1  OutDataTypeStr=boolean
  Data Type Conversion{1..5} (5 alike) : DataTypeConversion  OutDataTypeStr=double
  Display{1..6} (6 alike) : Display
  Divide{,1..4} (5 alike) : Product  Inputs=*/
  Integrator{,1..4} (5 alike) : Integrator
  tag scope: Comfort_time=global, ECO_time=global, EV_time=global, HEV_time=global, Sport_time=global
  wires:
  驾驶模式/1 -> Compare To Constant2/1, Compare To Constant1/1, Compare To Constant/1
  Compare To Constant/1 -> Data Type Conversion3/1
  Compare To Constant1/1 -> Data Type Conversion1/1
  Compare To Constant2/1 -> Data Type Conversion2/1
  Compare To Constant3/1 -> Data Type Conversion4/1
  能源模式/1 -> Display6/1, Compare To Constant3/1, Compare To Constant4/1
  Compare To Constant4/1 -> Data Type Conversion5/1
  Integrator/1 -> Divide/1
  Clock/1 -> Divide4/2, Divide3/2, Divide2/2, Divide1/2, Divide/2
  Divide/1 -> Display5/1, [ECO_time]
  Divide1/1 -> Display1/1, [Comfort_time]
  Divide2/1 -> Display2/1, [Sport_time]
  Divide3/1 -> Display3/1, [EV_time]
  Divide4/1 -> Display4/1, [HEV_time]
  Integrator1/1 -> Divide1/1
  Integrator2/1 -> Divide2/1
  Integrator3/1 -> Divide3/1
  Integrator4/1 -> Divide4/1
  Data Type Conversion3/1 -> Integrator/1
  Data Type Conversion1/1 -> Integrator1/1
  Data Type Conversion2/1 -> Integrator2/1
  Data Type Conversion4/1 -> Integrator3/1
  Data Type Conversion5/1 -> Integrator4/1

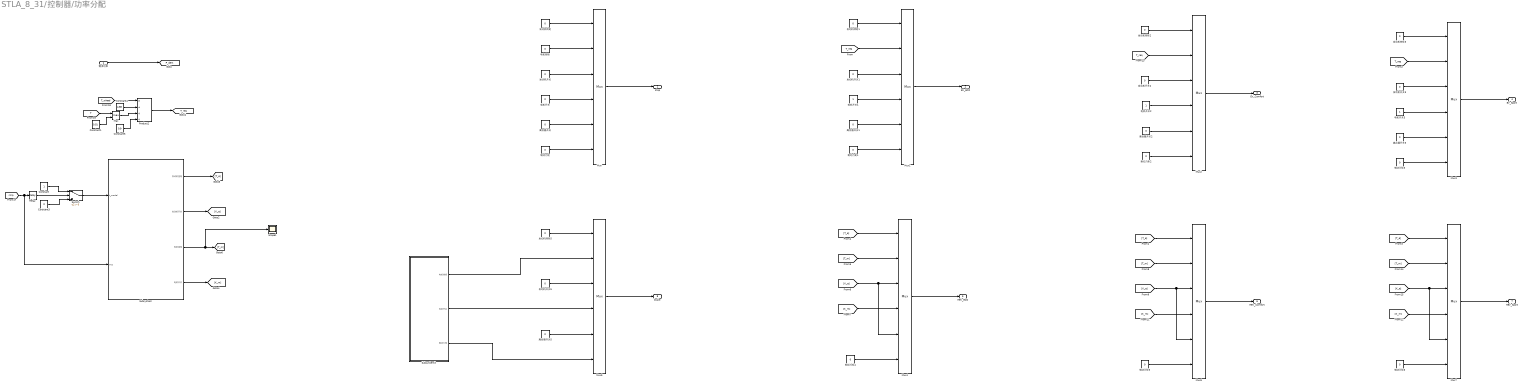
== system STLA_8_31/控制器/功率分配 ==
  需求功率 : Inport
  Constant : Constant
  Constant1 : Constant  Value=0.01
  Constant3 : Constant  Value=0
  Constant4 : Constant  Value=4.88
  Constant5 : Constant  Value=0.9
  Max : MinMax  Function=max  Inputs=2
  Mux{,1..7} (8 alike) : Mux  Inputs=6
  Product2 : Product  Inputs=*///
  Relay : Relay  OnSwitchValue=300  OffSwitchValue=150
  Scope1 : Scope
  Subsystem : Subsystem
  Subsystem3 : Subsystem
  Switch : Switch  Criteria=u2 > Threshold
  制动力矩{,1..6} (7 alike) : Constant  Value=0
  发动机开关{,1..3,5} (5 alike) : Constant  Value=0
  发动机转矩{,1..3,5} (5 alike) : Constant  Value=0
  电机开关 : Constant  Value=0
  电机开关1 : Constant
  电机开关2 : Constant
  电机开关3 : Constant
  电机转矩 : Constant  Value=0
  离合器开关{,1..3,5} (5 alike) : Constant  Value=0
  stop : Outport
  EV_ECO : Outport  Port=2
  EV_Comfort : Outport  Port=3
  EV_Sport : Outport  Port=4
  HEV_ECO : Outport  Port=5
  HEV_Comfort : Outport  Port=6
  HEV_Sport : Outport  Port=7
  brake : Outport  Port=8
  tag scope: P_dem=global, T_req=global
  wires:
  发动机转矩/1 -> Mux/1
  发动机开关/1 -> Mux/3
  电机转矩/1 -> Mux/2
  电机开关/1 -> Mux/4
  制动力矩/1 -> Mux/6
  离合器开关/1 -> Mux/5
  Mux/1 -> stop/1
  离合器开关1/1 -> Mux1/5
  Mux1/1 -> EV_ECO/1
  制动力矩1/1 -> Mux1/6
  发动机转矩1/1 -> Mux1/1
  发动机开关1/1 -> Mux1/3
  电机开关1/1 -> Mux1/4
  Mux4/1 -> HEV_ECO/1
  制动力矩4/1 -> Mux4/6
  Mux5/1 -> brake/1
  发动机转矩5/1 -> Mux5/1
  离合器开关5/1 -> Mux5/5
  发动机开关5/1 -> Mux5/3
  [T_req] -> Mux1/2
  发动机开关2/1 -> Mux2/3
  离合器开关2/1 -> Mux2/5
  制动力矩2/1 -> Mux2/6
  Mux2/1 -> EV_Comfort/1
  发动机转矩2/1 -> Mux2/1
  电机开关2/1 -> Mux2/4
  Mux3/1 -> EV_Sport/1
  制动力矩3/1 -> Mux3/6
  发动机转矩3/1 -> Mux3/1
  离合器开关3/1 -> Mux3/5
  电机开关3/1 -> Mux3/4
  发动机开关3/1 -> Mux3/3
  Mux6/1 -> HEV_Comfort/1
  Mux7/1 -> HEV_Sport/1
  [T_req] -> Mux2/2
  [T_req] -> Mux3/2
  Subsystem3/3("制动力矩 ") -> Mux5/6
  [K_m] -> Mux4/4
  [K_e] -> Mux4/5, Mux4/3
  制动力矩5/1 -> Mux6/6
  制动力矩6/1 -> Mux7/6
  [T_m] -> Mux4/2
  [T_e] -> Mux4/1
  Subsystem3/1(电机转矩) -> Mux5/2
  Subsystem3/2(电机开关) -> Mux5/4
  Subsystem/2(发动机开关) -> [K_e]
  Subsystem/4(电机开关) -> [K_m]
  [K_e] -> Mux6/5, Mux6/3
  [T_m] -> Mux6/2
  [T_e] -> Mux6/1
  [K_m] -> Mux6/4
  [K_m] -> Mux7/4
  [T_e] -> Mux7/1
  [T_m] -> Mux7/2
  [K_e] -> Mux7/5, Mux7/3
  需求功率/1 -> [P_dem]
  [rmp] -> Subsystem/2(rmp), Relay/1
  Relay/1 -> Switch/2
  Constant/1 -> Switch/1
  Constant3/1 -> Switch/3
  Switch/1 -> Subsystem/1(L_model)
  [T_wheel] -> Product2/1
  Constant4/1 -> Product2/2
  Constant5/1 -> Product2/4
  Product2/1 -> [T_req]
  Subsystem/1(发动机扭矩) -> [T_e]
  Subsystem/3(电机扭矩) -> Scope1/1, [T_m]
  [T] -> Max/1
  Max/1 -> Product2/3
  Constant1/1 -> Max/2

== system STLA_8_31/控制器/挡位切换 ==
  车速 : Inport
  油门开度 : Inport  Port=2
  制动开度 : Inport  Port=3
  Abs : Abs
  Abs1 : Abs
  Chart : Stateflow chart  TreatAsAtomicUnit=on
  Compare To Constant : simulink/Logic and Bit Operations/Compare To Constant  relop=<=  const=1e-4  OutDataTypeStr=boolean
  Compare To Constant1 : simulink/Logic and Bit Operations/Compare To Constant  relop=<=  const=1e-4  OutDataTypeStr=boolean
  Constant : Constant
  Data Type Conversion3 : DataTypeConversion  OutDataTypeStr=double
  Display1 : Display
  Integrator : Integrator  ExternalReset=either
  Product : Product
  Scope : Scope  NumInputPorts=2
  Scope1 : Scope
  Scope2 : Scope
  Scope3 : Scope
  Scope4 : Scope  NumInputPorts=2
  Out1 : Outport
  tag scope: POS_MONOSTABLE_LEVER=global
  wires:
  油门开度/1 -> Abs1/1
  Chart/2(ratio) -> Out1/1
  Chart/1(gear) -> [POS_MONOSTABLE_LEVER], Scope1/1, Display1/1
  制动开度/1 -> Abs/1
  车速/1 -> Chart/3(V)
  Data Type Conversion3/1 -> Integrator/1, Integrator/2
  Constant/1 -> Chart/4(PN_flag)
  Integrator/1 -> Scope2/1, Chart/5(T_ct)
  Compare To Constant/1 -> Scope4/2, Product/1
  Compare To Constant1/1 -> Scope/2, Product/2
  Product/1 -> Scope3/1, Data Type Conversion3/1
  Abs/1 -> Scope4/1, Chart/1(brake), Compare To Constant/1
  Abs1/1 -> Chart/2(throttle), Compare To Constant1/1, Scope/1

== system STLA_8_31/控制器/模式选择 ==
  油门信号 : Inport
  制动信号 : Inport  Port=2
  Chart : Stateflow chart  TreatAsAtomicUnit=on
      settings: PortSchema="{\"entries\":[{\"content\":{\"sides\":[{\"content\":{\"connectorIds\":[\"In3\",\"In4\",\"In1\",\"In2\"]},\"type\":\"ConnectorPlacement.EquallySpacedRectSide\",\"uuid\":\"a71f6391-e1d2-4931-91ac-1713c8a3738f\"},{\"content\":{\"connectorIds\":[\"Out1\"],\"side\":\"RIGHT\"},\"type\":\"ConnectorPlacement.EquallySpacedRectSide\",\"uuid\":\"fe57e218-1817-4c39-bfc1-b40cd5d4e9a9\"},{\"content\":{\"side\":\"TOP\"},\"type\":\"ConnectorPlacement.EquallySpacedRectSide\",\"uuid\":\"be5ec62b-3236-4b8b-9d89-5acfc240f42d\"}]},\"type\":\"ConnectorPlacement.EquallySpacedConnector\",\"uuid\":\"de164ca6-ce59-445c-bbbb-698006a1e93c\"}],\"packageUris\":[\"http://schema.mathworks.com/mf0/Connector/R2020b\"],\"version\":\"1.0\"}"
  Comfort : Constant
  EV1 : Constant  Value=0
  HEV1 : Constant
  Multiport Switch : MultiPortSwitch  DataPortOrder=Zero-based contiguous  DiagnosticForDefault=None  zeroidx=on
  Multiport Switch1 : MultiPortSwitch  DataPortOrder=Zero-based contiguous  Inputs=2  DiagnosticForDefault=None  zeroidx=on
  Scope : Scope
  Sport : Constant  Value=2
  eco : Constant  Value=0
  Model : Outport
  tag scope: STDE_DRV_DYN_MODE_STATE=global, STDE_DRV_ENGY_MODE_STATE=global
  wires:
  eco/1 -> Multiport Switch/2
  Comfort/1 -> Multiport Switch/3
  Sport/1 -> Multiport Switch/4
  [D_model] -> Multiport Switch/1
  Multiport Switch1/1 -> [STDE_DRV_ENGY_MODE_STATE], Chart/3(E_model)
  Multiport Switch/1 -> Chart/4(D_model), [STDE_DRV_DYN_MODE_STATE]
  油门信号/1 -> Chart/1(throttle)
  制动信号/1 -> Chart/2(brake)
  Chart/1(Model) -> Scope/1, Model/1
  HEV1/1 -> Multiport Switch1/3
  EV1/1 -> Multiport Switch1/2
  [E_model] -> Multiport Switch1/1

== system STLA_8_31/电机/Subsystem ==
  In1 : Inport
  Constant1 : Constant  Value=9550
  Constant2 : Constant  Value=9550
  Max : MinMax  Function=max  Inputs=2
  Min : MinMax  Inputs=2
  Product : Product
  Product1 : Product  Inputs=**/
  Product2 : Product  Inputs=***/
  峰值扭矩 : Lookup_n-D  NumberOfTableDimensions=1  BreakpointsForDimension1=rpm_M  Table=peak_torque_M  InternalRulePriority=Speed  RndMeth=Simplest  InputSameDT=on
  持续转矩 : Lookup_n-D  NumberOfTableDimensions=1  BreakpointsForDimension1=rpm_M  Table=continuous_torque_M  InternalRulePriority=Speed  RndMeth=Simplest  InputSameDT=on
  tag scope: Pm_lim=global, Tm_lim=global
  wires:
  In1/1 -> 峰值扭矩/1, 持续转矩/1
  持续转矩/1 -> Max/2
  [T_derate] -> Product/2
  Product/1 -> Max/1
  Constant2/1 -> Product1/3
  [rmp] -> Product1/1
  Product1/1 -> Min/2
  Constant1/1 -> Product2/4
  [rmp] -> Product2/1
  峰值扭矩/1 -> Product/1, Product2/2
  Product2/1 -> Min/1
  Min/1 -> [Pm_lim]
  Max/1 -> [Tm_lim], Product1/2
  [P_derate] -> Product2/3

== system STLA_8_31/电机/Subsystem1 ==
  转矩 : Inport
  转速 : Inport  Port=2
  " " : Constant  Value=9550
  " 1" : Constant  Value=9550
  2-D Lookup Table : Lookup_n-D  BreakpointsForDimension1=eff_torques  BreakpointsForDimension2=eff_speeds  Table=m_eff  InternalRulePriority=Speed  RndMeth=Simplest  InputSameDT=on
      settings: InputPortMap=u0,u1
  Constant : Constant  Value=0.05
  Gain2 : Gain  Gain=-1
  Max : MinMax  Function=max  Inputs=2
  Product : Product  Inputs=**//
  Product2 : Product  Inputs=***/
  Saturation Dynamic3 : simulink/Discontinuities/Saturation Dynamic  OutMin=[]  OutMax=[]  OutDataTypeStr=Inherit: Same as second input  OutDataType=fixdt(1, 16)  OutScaling=2^-10  DoSatur=off
  效率1 : Constant  Value=0.9
  电机输出转矩 : Outport
  Out1 : Outport  Port=2
  Out2 : Outport  Port=3
  wires:
  2-D Lookup Table/1 -> Max/2, Product2/3
  " "/1 -> Product/4
  " 1"/1 -> Product2/4
  转矩/1 -> 2-D Lookup Table/2, Saturation Dynamic3/2, Product/1, Product2/1
  转速/1 -> 2-D Lookup Table/1, Product2/2, Product/2
  Product2/1 -> Out2/1
  Product/1 -> Out1/1
  Constant/1 -> Max/1
  Max/1 -> Product/3
  Saturation Dynamic3/1 -> 电机输出转矩/1
  [Tm_lim] -> Gain2/1, Saturation Dynamic3/1
  Gain2/1 -> Saturation Dynamic3/3

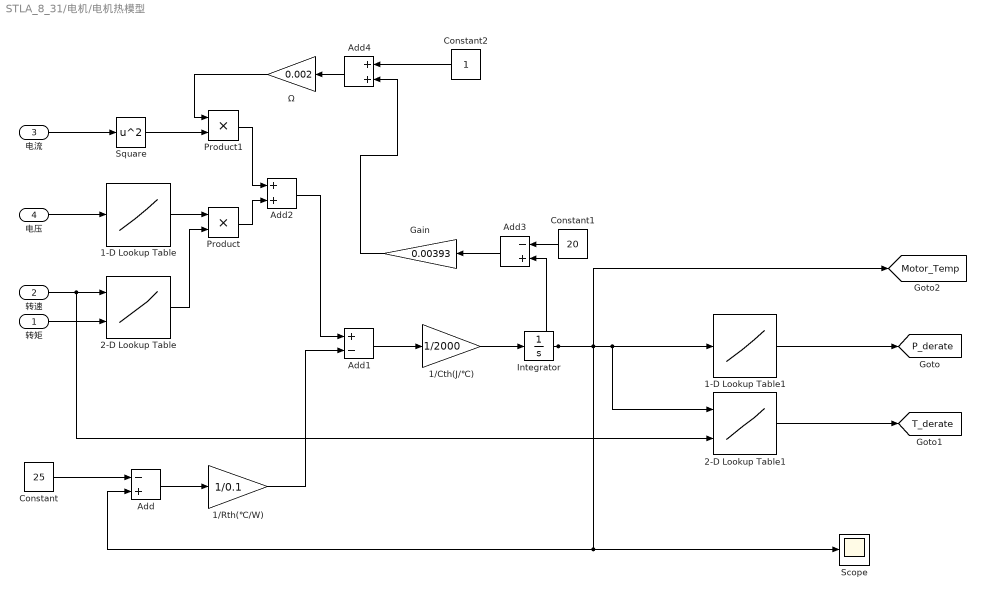
== system STLA_8_31/电机/电机热模型 ==
  转矩 : Inport
  转速 : Inport  Port=2
  电流 : Inport  Port=3
  电压 : Inport  Port=4
  1-D Lookup Table : Lookup_n-D  NumberOfTableDimensions=1  BreakpointsForDimension1=[280, 310, 340, 380, 420]  Table=[1.25, 1.15, 1.05, 1.00, 0.95]  InternalRulePriority=Speed  RndMeth=Simplest  InputSameDT=on
  1-D Lookup Table1 : Lookup_n-D  NumberOfTableDimensions=1  BreakpointsForDimension1=[20 100 120 140 150 160]  Table=|  InternalRulePriority=Speed  RndMeth=Simplest  InputSameDT=on
      | [
      | 1
      | 1
      | 0.95
      | 0.8
      | 0.6
      | 0
      | ]
  1/Cth(J/℃) : Gain  Gain=1/2000
  1/Rth(℃/W) : Gain  Gain=1/0.1
  2-D Lookup Table : Lookup_n-D  BreakpointsForDimension1=speed_bp  BreakpointsForDimension2=torque_bp  Table=Padd  InternalRulePriority=Speed  RndMeth=Simplest  InputSameDT=on
      settings: InputPortMap=u0,u1
  2-D Lookup Table1 : Lookup_n-D  BreakpointsForDimension1=[20 80 120 140 160]  BreakpointsForDimension2=[0 1000 2000 3000 4000 5000 6000]  Table=|  InternalRulePriority=Speed  RndMeth=Simplest  InputSameDT=on
      | [
      | 1    1    1    1    1    1    1;
      | 1    1    1    1    1    1    1;
      | 0.9  0.9  0.85 0.8  0.75 0.7  0.6;
      | 0.7  0.65 0.6  0.55 0.5  0.45 0.4;
      | 0    0    0    0    0    0    0
      | ]
      settings: InputPortMap=u0,u1
  Add : Sum  Inputs=-+
  Add1 : Sum  Inputs=+-
  Add2 : Sum
  Add3 : Sum  Inputs=-+
  Add4 : Sum
  Constant : Constant  Value=25
  Constant1 : Constant  Value=20
  Constant2 : Constant
  Gain : Gain  Gain=0.00393
  Integrator : Integrator  InitialCondition=25
  Product : Product
  Product1 : Product
  Scope : Scope
  Square : Math  Operator=square  SaturateOnIntegerOverflow=on
  Ω : Gain  Gain=0.002
  tag scope: Motor_Temp=global, P_derate=global, T_derate=global
  wires:
  电流/1 -> Square/1
  Square/1 -> Product1/2
  转速/1 -> 2-D Lookup Table1/2, 2-D Lookup Table/1
  转矩/1 -> 2-D Lookup Table/2
  电压/1 -> 1-D Lookup Table/1
  Add/1 -> 1/Rth(℃/W)/1
  1/Rth(℃/W)/1 -> Add1/2
  Add1/1 -> 1/Cth(J/℃)/1
  1/Cth(J/℃)/1 -> Integrator/1
  Constant/1 -> Add/1
  1-D Lookup Table1/1 -> [P_derate]
  1-D Lookup Table/1 -> Product/1
  2-D Lookup Table/1 -> Product/2
  Product1/1 -> Add2/1
  Product/1 -> Add2/2
  Add2/1 -> Add1/1
  Constant1/1 -> Add3/1
  Add3/1 -> Gain/1
  Gain/1 -> Add4/2
  Constant2/1 -> Add4/1
  Add4/1 -> Ω/1
  Ω/1 -> Product1/1
  Integrator/1 -> Add3/2, Scope/1, Add/2, [Motor_Temp], 2-D Lookup Table1/1, 1-D Lookup Table1/1
  2-D Lookup Table1/1 -> [T_derate]

== system STLA_8_31/电池/Subsystem ==
  电流 : Inport
  " " : Gain  Gain=10
  Clock : Clock
  Constant : Constant  Value=0.01
  Constant1 : Constant  Value=25
  Divide : Product  Inputs=*/
  Gain1 : Gain  Gain=1/117000
  Integrator : Integrator  InitialCondition=25
  Integrator1 : Integrator
  Max : MinMax  Function=max  Inputs=2
  Memory : Memory
  Min : MinMax  Function=max  Inputs=2
  Saturation : Saturate  UpperLimit=190  LowerLimit=-40
  Square : Math  Operator=square  SaturateOnIntegerOverflow=on
  Sum : Sum  Inputs=|+-
  Sum1 : Sum  Inputs=|+-
  总内阻 : Gain  Gain=0.54
  实时温度 : Outport
  平均温度 : Outport  Port=2
  最高温度 : Outport  Port=3
  wires:
  Square/1 -> 总内阻/1
  Sum/1 -> " "/1
  总内阻/1 -> Sum1/1
  " "/1 -> Sum1/2
  Sum1/1 -> Gain1/1
  Gain1/1 -> Integrator/1
  Integrator/1 -> Saturation/1
  Saturation/1 -> Integrator1/1, Max/1, 实时温度/1, Sum/1
  Constant1/1 -> Sum/2
  电流/1 -> Square/1
  Integrator1/1 -> Divide/1
  Divide/1 -> 平均温度/1
  Memory/1 -> Max/2
  Max/1 -> Memory/1, 最高温度/1
  Clock/1 -> Min/1
  Constant/1 -> Min/2
  Min/1 -> Divide/2

== system STLA_8_31/后处理/Subsystem/Triggered Subsystem ==
  In1 : Inport
  Trigger : TriggerPort  VariantControl=(inherit)
  Out1 : Outport
  wires:
  In1/1 -> Out1/1

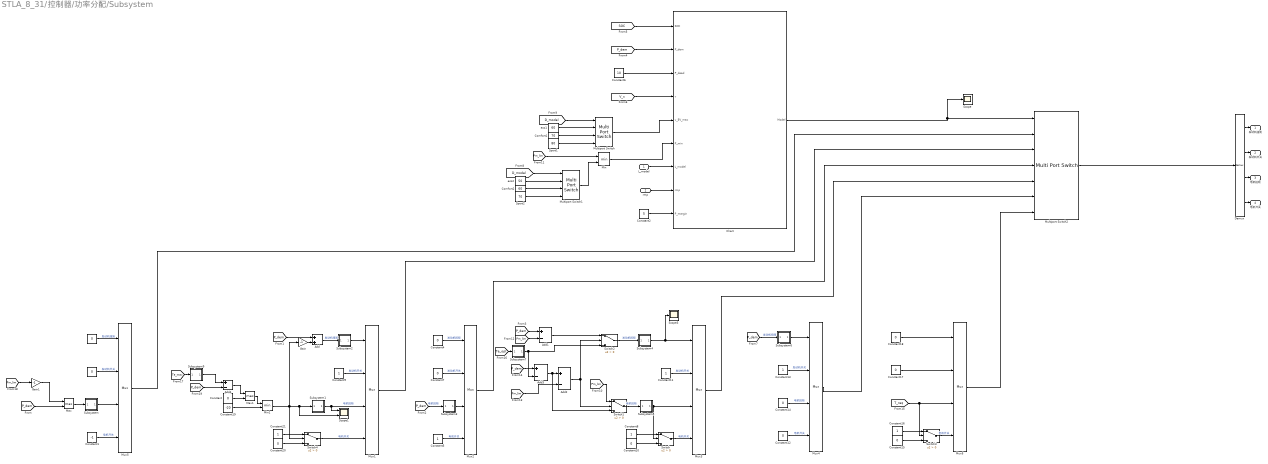
== system STLA_8_31/控制器/功率分配/Subsystem ==
  L_model : Inport
  rmp : Inport  Port=2
  " " : Constant  Value=0
  "   " : Constant  Value=0
  Add : Sum
  Add{1..4} (4 alike) : Sum  Inputs=+-
  Chart : Stateflow chart  TreatAsAtomicUnit=on
  Comfort1 : Constant  Value=70
  Comfort2 : Constant  Value=60
  Constant{,4,7,10,12,14..15,17..18,20} (10 alike) : Constant  Value=0
  Constant1 : Constant  Value=-1
  Constant{5,8..9,11,13,16,21} (7 alike) : Constant
  Constant19 : Constant  Value=-20
  Constant2 : Constant  Value=5
  Constant6 : Constant  Value=10
  Demux : Demux
  Gain : Gain  Gain=-1
  Gain1 : Gain  Gain=-1
  Max : MinMax  Function=max  Inputs=2
  Max1 : MinMax  Function=max  Inputs=2
  Min : MinMax  Inputs=2
  Min1 : MinMax  Inputs=2
  Multiport Switch : MultiPortSwitch  DataPortOrder=Zero-based contiguous  zeroidx=on
  Multiport Switch1 : MultiPortSwitch  DataPortOrder=Zero-based contiguous  zeroidx=on
  Multiport Switch2 : MultiPortSwitch  Inputs=6
  Mux{1..6} (6 alike) : Mux
  Scope : Scope
  Scope1 : Scope  NumInputPorts=2
  Scope3 : Scope
  Sport1 : Constant  Value=80
  Sport2 : Constant  Value=70
  Subsystem : Subsystem
  Subsystem1 : Subsystem
  Subsystem2 : Subsystem
  Subsystem3 : Subsystem
  Subsystem4 : Subsystem
  Subsystem5 : Subsystem
  Subsystem6 : Subsystem
  Subsystem7 : Subsystem
  Subsystem9 : Subsystem
  Switch{,1..4} (5 alike) : Switch  Criteria=u2 > Threshold
  eco1 : Constant  Value=60
  eco2 : Constant  Value=50
  发动机扭矩 : Outport
  发动机开关 : Outport  Port=2
  电机扭矩 : Outport  Port=3
  电机开关 : Outport  Port=4
  wires:
  [D_model] -> Multiport Switch1/1
  Comfort2/1 -> Multiport Switch1/3
  Min/1 -> Chart/6(P_min)
  [SOC] -> Chart/1(SOC)
  Sport2/1 -> Multiport Switch1/4
  eco2/1 -> Multiport Switch1/2
  Demux/1 -> 发动机扭矩/1
  Multiport Switch2/1 -> Demux/1
  Constant6/1 -> Chart/3(P_dead)
  eco1/1 -> Multiport Switch/2
  Multiport Switch/1 -> Chart/5(v_EV_max)
  Sport1/1 -> Multiport Switch/4
  [D_model] -> Multiport Switch/1
  [V_x] -> Chart/4(v)
  Multiport Switch1/1 -> Min/2
  Comfort1/1 -> Multiport Switch/3
  Demux/2 -> 发动机开关/1
  [Pm_lim] -> Min/1
  Chart/1(Model) -> Scope/1, Multiport Switch2/1
  Demux/3 -> 电机扭矩/1
  Demux/4 -> 电机开关/1
  " "/1 -> Mux5/1  "发动机扭矩"
  "   "/1 -> Mux5/2  "发动机开关"
  Constant1/1 -> Mux5/4  "电机开关"
  [Pm_lim] -> Gain1/1
  [P_dem] -> Max/2
  Min1/1 -> Gain/1, Switch4/2, Subsystem1/1(In1), Scope1/2
  Constant9/1 -> Mux1/2  "发动机开关"
  Add/1 -> Subsystem2/1(In1)  "发动机扭矩"
  [P_dem] -> Add/1
  Gain/1 -> Add/2
  Constant4/1 -> Mux2/1  "发动机扭矩"
  Constant7/1 -> Mux2/2  "发动机开关"
  [P_dem] -> Subsystem3/1(In1)  "电机扭矩"
  Constant5/1 -> Mux2/4  "电机开关"
  Switch/1 -> Mux3/4  "电机开关"
  Switch1/1 -> Subsystem5/1(In1)  "电机扭矩"
  Constant11/1 -> Mux3/2  "发动机开关"
  Switch2/1 -> Subsystem4/1(In1)  "发动机扭矩"
  [P_dem] -> Subsystem6/1(In1)  "发动机扭矩"
  Constant13/1 -> Mux4/2  "发动机开关"
  Constant14/1 -> Mux4/3  "电机扭矩"
  Constant12/1 -> Mux4/4  "电机开关"
  Constant8/1 -> Switch/1
  Constant10/1 -> Switch/3
  Mux5/1 -> Multiport Switch2/2
  Mux1/1 -> Multiport Switch2/3
  Mux2/1 -> Multiport Switch2/4
  Mux3/1 -> Multiport Switch2/5
  Mux4/1 -> Multiport Switch2/6
  Add2/1 -> Switch1/2, Switch2/2
  [Pm_lim] -> Switch1/1
  [P_dem] -> Add3/1
  [Te_opt] -> Subsystem7/1(In1)
  Add3/1 -> Switch1/3, Add2/1
  [Pm_lim] -> Add2/2
  [Pm_lim] -> Add1/2
  [P_dem] -> Add1/1
  Add1/1 -> Switch2/1
  L_model/1 -> Chart/7(L_model)
  Max/1 -> Subsystem/1(In1)
  Subsystem/1(Out1) -> Mux5/3
  Subsystem1/1(Out1) -> Scope1/1, Mux1/3  "电机扭矩"
  Subsystem2/1(Out1) -> Mux1/1
  Subsystem3/1(Out1) -> Mux2/3
  Subsystem5/1(Out1) -> Switch/2, Mux3/3
  Subsystem6/1(Out1) -> Mux4/1
  Mux6/1 -> Multiport Switch2/7
  [T_req] -> Switch3/2, Mux6/3
  Constant15/1 -> Switch3/3
  Constant16/1 -> Switch3/1
  Switch3/1 -> Mux6/4  "电机开关"
  Constant17/1 -> Mux6/2
  Constant18/1 -> Mux6/1
  rmp/1 -> Chart/8(rmp)
  [Te_max] -> Subsystem9/1(In1)
  Subsystem9/1(Out1) -> Add4/1
  [P_dem] -> Add4/2
  Constant/1 -> Max1/2
  Add4/1 -> Max1/1
  Max1/1 -> Min1/1
  Constant19/1 -> Min1/2
  Constant20/1 -> Switch4/3
  Constant21/1 -> Switch4/1
  Switch4/1 -> Mux1/4  "电机开关"
  Gain1/1 -> Max/1
  Constant2/1 -> Chart/9(P_margin)
  [P_dem] -> Chart/2(P_dem)
  Subsystem7/1(Out1) -> Switch2/3, Add3/2
  Subsystem4/1(Out1) -> Scope3/1, Mux3/1

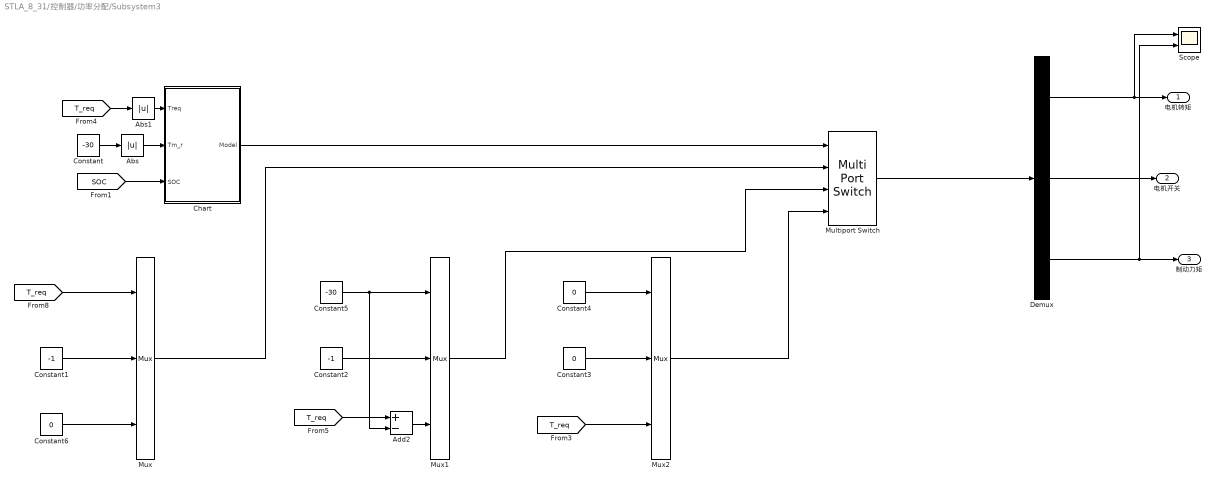
== system STLA_8_31/控制器/功率分配/Subsystem3 ==
  Abs : Abs
  Abs1 : Abs
  Add2 : Sum  Inputs=+-
  Chart : Stateflow chart  TreatAsAtomicUnit=on
  Constant : Constant  Value=-30
  Constant1 : Constant  Value=-1
  Constant2 : Constant  Value=-1
  Constant3 : Constant  Value=0
  Constant4 : Constant  Value=0
  Constant5 : Constant  Value=-30
  Constant6 : Constant  Value=0
  Demux : Demux  Outputs=3
  Multiport Switch : MultiPortSwitch
  Mux : Mux  Inputs=3
  Mux1 : Mux  Inputs=3
  Mux2 : Mux  Inputs=3
  Scope : Scope  NumInputPorts=2
  电机转矩 : Outport
  电机开关 : Outport  Port=2
  "制动力矩 " : Outport  Port=3
  wires:
  Multiport Switch/1 -> Demux/1
  Mux/1 -> Multiport Switch/2
  Chart/1(Model) -> Multiport Switch/1
  Demux/3 -> Scope/2, "制动力矩 "/1
  Demux/2 -> 电机开关/1
  Demux/1 -> Scope/1, 电机转矩/1
  [T_req] -> Abs1/1
  Constant/1 -> Abs/1
  [SOC] -> Chart/3(SOC)
  [T_req] -> Mux/1
  Constant1/1 -> Mux/2
  Constant6/1 -> Mux/3
  Constant5/1 -> Mux1/1, Add2/2
  Constant2/1 -> Mux1/2
  Add2/1 -> Mux1/3
  [T_req] -> Add2/1
  [T_req] -> Mux2/3
  Constant3/1 -> Mux2/2
  Constant4/1 -> Mux2/1
  Mux1/1 -> Multiport Switch/3
  Mux2/1 -> Multiport Switch/4
  Abs/1 -> Chart/2(Tm_r)
  Abs1/1 -> Chart/1(Treq)

== system STLA_8_31/控制器/功率分配/Subsystem/Subsystem ==
  In1 : Inport
  Constant : Constant
  Constant15 : Constant  Value=9550
  Max : MinMax  Function=max  Inputs=2
  Product1 : Product  Inputs=**/
  Out1 : Outport
  wires:
  Constant15/1 -> Product1/2
  Product1/1 -> Out1/1
  In1/1 -> Product1/1
  [rmp] -> Max/1
  Max/1 -> Product1/3
  Constant/1 -> Max/2

== system STLA_8_31/控制器/功率分配/Subsystem/Subsystem1 ==
  In1 : Inport
  Constant : Constant
  Constant15 : Constant  Value=9550
  Max : MinMax  Function=max  Inputs=2
  Product1 : Product  Inputs=**/
  Out1 : Outport
  wires:
  Constant15/1 -> Product1/2
  Product1/1 -> Out1/1
  In1/1 -> Product1/1
  [rmp] -> Max/1
  Max/1 -> Product1/3
  Constant/1 -> Max/2

== system STLA_8_31/控制器/功率分配/Subsystem/Subsystem2 ==
  In1 : Inport
  Constant : Constant
  Constant15 : Constant  Value=9550
  Max : MinMax  Function=max  Inputs=2
  Product1 : Product  Inputs=**/
  Out1 : Outport
  wires:
  Constant15/1 -> Product1/2
  Product1/1 -> Out1/1
  In1/1 -> Product1/1
  [rmp] -> Max/1
  Max/1 -> Product1/3
  Constant/1 -> Max/2

== system STLA_8_31/控制器/功率分配/Subsystem/Subsystem3 ==
  In1 : Inport
  Constant : Constant
  Constant15 : Constant  Value=9550
  Max : MinMax  Function=max  Inputs=2
  Product1 : Product  Inputs=**/
  Out1 : Outport
  wires:
  Constant15/1 -> Product1/2
  Product1/1 -> Out1/1
  In1/1 -> Product1/1
  [rmp] -> Max/1
  Max/1 -> Product1/3
  Constant/1 -> Max/2

== system STLA_8_31/控制器/功率分配/Subsystem/Subsystem4 ==
  In1 : Inport
  Constant : Constant
  Constant15 : Constant  Value=9550
  Max : MinMax  Function=max  Inputs=2
  Product1 : Product  Inputs=**/
  Out1 : Outport
  wires:
  Constant15/1 -> Product1/2
  Product1/1 -> Out1/1
  In1/1 -> Product1/1
  [rmp] -> Max/1
  Max/1 -> Product1/3
  Constant/1 -> Max/2

== system STLA_8_31/控制器/功率分配/Subsystem/Subsystem5 ==
  In1 : Inport
  Constant : Constant
  Constant15 : Constant  Value=9550
  Max : MinMax  Function=max  Inputs=2
  Product1 : Product  Inputs=**/
  Out1 : Outport
  wires:
  Constant15/1 -> Product1/2
  Product1/1 -> Out1/1
  In1/1 -> Product1/1
  [rmp] -> Max/1
  Max/1 -> Product1/3
  Constant/1 -> Max/2

== system STLA_8_31/控制器/功率分配/Subsystem/Subsystem6 ==
  In1 : Inport
  Constant : Constant
  Constant15 : Constant  Value=9550
  Max : MinMax  Function=max  Inputs=2
  Product1 : Product  Inputs=**/
  Out1 : Outport
  wires:
  Constant15/1 -> Product1/2
  Product1/1 -> Out1/1
  In1/1 -> Product1/1
  [rmp] -> Max/1
  Max/1 -> Product1/3
  Constant/1 -> Max/2

== system STLA_8_31/控制器/功率分配/Subsystem/Subsystem7 ==
  In1 : Inport
  Constant : Constant
  Constant15 : Constant  Value=9550
  Max : MinMax  Function=max  Inputs=2
  Product1 : Product  Inputs=*/*
  Out1 : Outport
  wires:
  Constant15/1 -> Product1/2
  Product1/1 -> Out1/1
  In1/1 -> Product1/1
  [rmp] -> Max/1
  Max/1 -> Product1/3
  Constant/1 -> Max/2

== system STLA_8_31/控制器/功率分配/Subsystem/Subsystem9 ==
  In1 : Inport
  Constant : Constant
  Constant15 : Constant  Value=9550
  Max : MinMax  Function=max  Inputs=2
  Product1 : Product  Inputs=*/*
  Out1 : Outport
  wires:
  Constant15/1 -> Product1/2
  Product1/1 -> Out1/1
  In1/1 -> Product1/1
  [rmp] -> Max/1
  Max/1 -> Product1/3
  Constant/1 -> Max/2

== stateflow chart STLA_8_31/控制器/功率分配/Subsystem/Chart ==
  state Charge
    entry:
    Model=2;
  state Coast
    entry:
    Model=1;
  state EV
    entry:
    Model=3;
  state Low_speed
    entry:
    Model=6;
  state Hybrid1
    entry:
    Model=4;
  state Engine
    entry:
    Model=5;
  Charge -> (junction 44) : [SOC>0.45 | L_model==0 | rmp<1500]
  (junction 44) -> Charge [order 2] : [SOC<0.35 & P_dem>P_dead&L_model==1&rmp>1500]
  (junction 44) -> Coast [order 1] : [P_dem<-P_dead]
  (junction 44) -> EV [order 3] : [SOC > 0.5 & P_dem < (P_min - P_margin) & v < v_EV_max & L_model==1]
  Coast -> (junction 44) : [(P_dem<-P_dead)==0 | L_model==0]
  EV -> (junction 44) : [SOC < 0.4| P_dem > P_min | v > v_EV_max | L_model==0]
  (junction 44) -> Low_speed [order 6] : [L_model==0]
  (junction 44) -> Hybrid1 [order 4] : [P_dem>P_min &SOC>0.25&L_model==1]
  Low_speed -> (junction 44) : [L_model==1]
  Hybrid1 -> (junction 44) : [[(P_dem < (P_min - P_margin)) | (SOC <= 0.25) | L_model==0]]
  (junction 44) -> Engine [order 5] : [P_dem>P_dead&L_model==1]
  Engine -> (junction 44) : [P_dem<P_dead | L_model==0 |(P_dem>P_min &SOC>0.25)]
  (default) -> Engine
  data: Model output; SOC input; P_dem input; P_dead input; v input; v_EV_max input; P_min input; L_model input; rmp input; P_margin input

== stateflow chart STLA_8_31/控制器/挡位切换/Chart ==
  state D
    state D1
      entry:
      ratio=3.8;
      gear=2;
    state D2
      entry:
      ratio=2.2;
      gear=3;
    state D3
      entry:
      ratio=1.4;
      gear=4;
    state D4
      entry:
      ratio=1;
      gear=5;
    state D5
      entry:
      ratio=0.8;
      gear=6;
    state D6
      entry:
      ratio=0.7;
      gear=7;
    state D7
      entry:
      ratio=0.6;
      gear=8;
    (default) -> D1
    D2 -> D3 [order 1] : [V>=25]
    D3 -> D4 [order 2] : [V>=40]
    D4 -> D5 [order 2] : [V>=55]
    D5 -> D6 [order 2] : [V>=75]
    D1 -> D2 : [V>=15]
    D6 -> D7 [order 2] : [V>=100]
    D5 -> D4 [order 1] : [V<=45]
    D7 -> D6 : [V<=70]
    D4 -> D3 [order 1] : [V<=30]
    D3 -> D2 [order 1] : [V<=20]
    D6 -> D5 [order 1] : [V<=70]
    D2 -> D1 [order 2] : [V<=12]
  state P_N
    state P
      entry:
      gear=0;
    state N
      entry:
      gear=1;
    (default) -> P
    P -> N : [PN_flag==0]
    N -> P : [PN_flag==1]
  (default) -> P_N
  P_N -> D : [throttle>1e-4|brake>1e-4]
  D -> P_N : [throttle<1e-4&brake<1e-4&T_ct>=20]
  data: brake input; throttle input; gear output; ratio output; V input; PN_flag input; T_ct input
